simulink model "inputs_version"  (R2022a)
settings: Solver=VariableStepAuto  StartTime=0.0  StopTime=20  RelTol=1e-3
undefined symbols (not defined in the file or in its folder): sigbuilder_block
libraries: dspsrcs4 x1

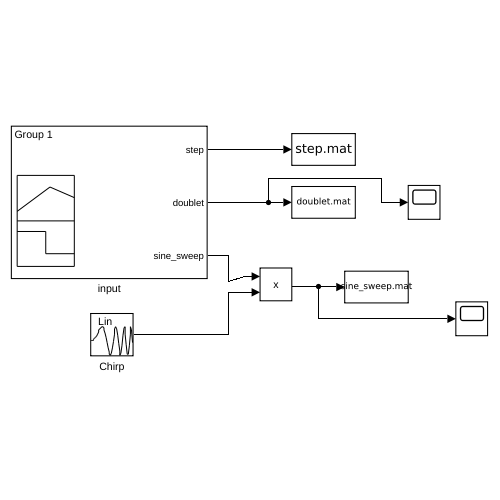
[thumbnail: Simulink's stored preview of the top-level diagram]
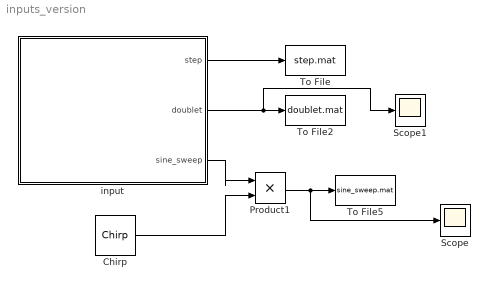
== system inputs_version ==
  Chirp : dspsrcs4/Chirp  sweep=Linear  mode=Unidirectional  f0=0  f1=3  t1=20  Tsweep=20  phase=0  Ts=0.02  spf=1  datatype=Double  OutputFrames=off
  Product1 : Product
  Scope : Scope
  Scope1 : Scope
  To File : ToFile  Filename=step.mat  MatrixName=step  SaveFormat=Timeseries  SampleTime=0.02
  To File2 : ToFile  Filename=doublet.mat  MatrixName=doublet  SaveFormat=Timeseries  SampleTime=0.02
  To File5 : ToFile  Filename=sine_sweep.mat  MatrixName=sine_sweep  SaveFormat=Timeseries  SampleTime=0.02
  input : Subsystem  Tag=STV Subsys  LoadFcn=sigbuilder_block('load');  StartFcn=sigbuilder_block('start');  StopFcn=sigbuilder_block('stop');  ClipboardFcn=sigbuilder_block('clipboard');  mask(Sigbuilder block){tuvar=[0:10]}
      mask help: Simulink:masks:SigbuilderBlock_MD
      mask init:
      | if ~strcmp(get_param(bdroot(gcbh),'SimulationStatus'),'stopped') tuvar = sigbuilder_block('maskInit'); end
  wires:
  input/1(step) -> To File/1
  input/2(doublet) -> Scope1/1, To File2/1
  input/3(sine_sweep) -> Product1/1
  Chirp/1 -> Product1/2
  Product1/1 -> Scope/1, To File5/1

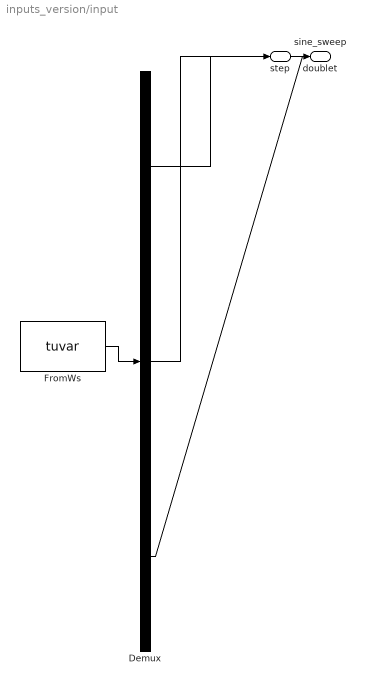
== system inputs_version/input ==
  Demux : Demux  Tag=STV Demux  Outputs=3
  FromWs : FromWorkspace  Tag=STV FromWs  VariableName=tuvar  SampleTime=1/50
      SigBuilderData=|
      | common.afterFinalStr = 'Extrapolate'
      | common.sampleTime = '1/50'
      | dataSet.timeRange = [0 20]
      | dataSet.name = 'Group 1'
      | sbobj.Groups.Name = 'Group 1'
      | sbobj.Groups.Signals(1).Name = 'step'
      | sbobj.Groups.Signals(1).XData = [0 1.98 1.98 5.02 20]
      | sbobj.Groups.Signals(1).YData = [0 0 0.1 0.1 0.1]
      | sbobj.Groups.Signals(2).Name = 'doublet'
      | sbobj.Groups.Signals(2).XData = [0 2 2 2.52 2.52 2.98 2.98 20]
      | sbobj.Groups.Signals(2).YData = [0 0 0.1 0.1 -0.1 -0.1 0 0]
      | sbobj.Groups.Signals(3).Name = 'sine_sweep'
      | sbobj.Groups.Signals(3).XData = [0 1.98 1.98 20]
      | sbobj.Groups.Signals(3).YData = [0 0 0.1 0.1]
      | sbobj.Groups.TimeRange = [0 20]
  step : Outport  Tag=STV Outport
  doublet : Outport  Tag=STV Outport  Port=2
  sine_sweep : Outport  Tag=STV Outport  Port=3
  wires:
  Demux/1 -> step/1
  FromWs/1 -> Demux/1
  Demux/2 -> doublet/1
  Demux/3 -> sine_sweep/1
